simulink model "controller"  (Simulink 8.6)
settings: Solver=FixedStepDiscrete  StartTime=0.0  StopTime=inf  FixedStep=Ts  RelTol=1e-3
InitFcn:
  | initTrqBalancingSeeSaw;
values from neighbouring files (symbols this model uses):
  directionOfOscillation = [0;1;0]    [init.m]
  noOscillationTime = 0    [init.m]
  referenceParams = [0.00  0.1]    [init.m]
  ROBOT_DOF = 23    [init.m]
  seesaw = struct    [init.m]
undefined symbols (not defined in the file or in its folder): bVectorConstraints, CONFIG, ConstraintsMatrix, footSize, gain, LEFT_RIGHT_FOOT_IN_CONTACT, reg, sat
libraries: WBToolboxLibrary x29, WBCLibrary x12, simulink x2
settings Model: Creator=makaveli  LastModifiedBy=DanielePucci
settings DataIOCC: SignalLoggingSaveFormat=Dataset
settings OptimizationCC: ExpressionDepthLimit=128
settings DebuggingCC: UnderspecifiedInitializationDetection=Simplified  MergeDetectMultiDrivingBlocksExec=error  FcnCallInpInsideContextMsg=EnableAllAsError  StateNameClashWarn=none
settings GRTTargetCC: CombineOutputUpdateFcns=on  GRTInterface=off
settings ConfigComp: CovSFcnEnable=off

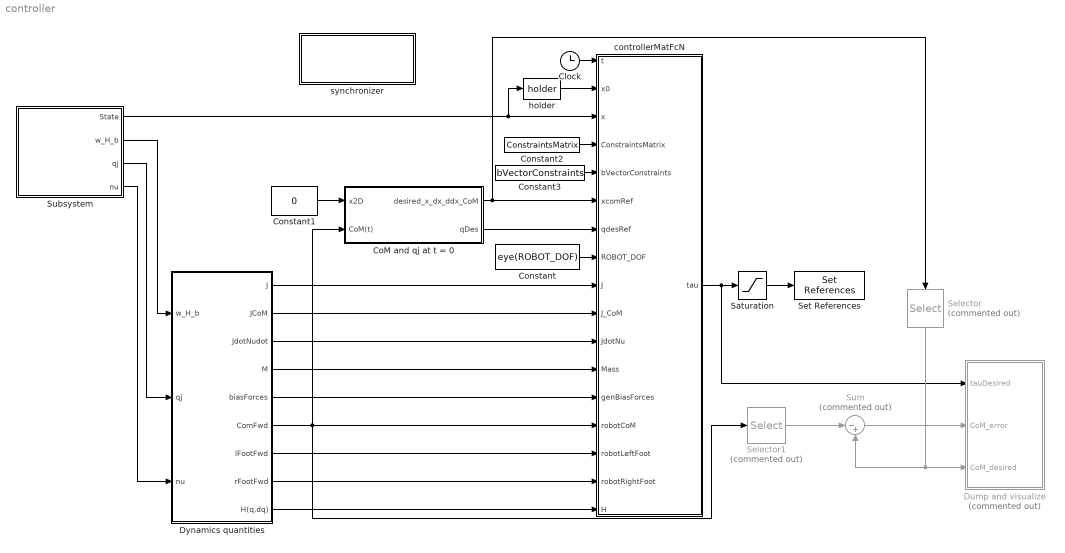
== system controller ==
  Clock : Clock
  CoM and qj at t = 0 : Subsystem  Priority=2
  Constant : Constant  Value=eye(ROBOT_DOF)
  Constant1 : Constant  Value=0
  Constant2 : Constant  Value=ConstraintsMatrix
  Constant3 : Constant  Value=bVectorConstraints
  Dump and visualize : Subsystem  Commented=on
  Dynamics quantities : Subsystem  Priority=3
  Saturation : Saturate  UpperLimit=sat.torque  LowerLimit=-sat.torque
  Selector : Selector  Commented=on  NumberOfDimensions=2  InputPortWidth=3  IndexOptions=Index vector (dialog),Index vector (dialog)  Indices=[1:3],1  OutputSizes=1,1
  Selector1 : Selector  Commented=on  InputPortWidth=7  IndexOptions=Index vector (dialog)  Indices=[1:3]  OutputSizes=1
  Set References : WBToolboxLibrary/wholeBodyActuators/Set References  controlType=Torque  robotName=WBT_robotName  localName=WBT_modelName  wbiFile=WBT_wbiFilename  wbiList=WBT_wbiList
  Subsystem : Subsystem  Priority=1
      mask Display:
      | disp('State');
      | port_label('output',1,'x')
      | port_label('output',2,'w_H_b')
      | port_label('output',3,'q_j')
      | port_label('output',4,'nu')
  Sum : Sum  Commented=on  Inputs=|-+
  controllerMatFcN : MATLAB Function  TreatAsAtomicUnit=on
  "holder " : WBToolboxLibrary/Utilities/holder 
  synchronizer : Subsystem
      mask Display: disp('SYNCHRONIZER')
  wires:
  Clock/1 -> controllerMatFcN/1(t)
  Subsystem/1(State) -> "holder "/1, controllerMatFcN/3(x)
  Subsystem/4(nu) -> Dynamics quantities/3(nu)
  CoM and qj at t = 0/1(desired_x_dx_ddx_CoM) -> Selector/1, controllerMatFcN/6(xcomRef)
  CoM and qj at t = 0/2(qDes) -> controllerMatFcN/7(qdesRef)
  Constant/1 -> controllerMatFcN/8(ROBOT_DOF)
  Dynamics quantities/1(J) -> controllerMatFcN/9(J)
  Dynamics quantities/2(JCoM) -> controllerMatFcN/10(J_CoM)
  Dynamics quantities/3(JdotNudot) -> controllerMatFcN/11(JdotNu)
  Dynamics quantities/4(M) -> controllerMatFcN/12(Mass)
  Dynamics quantities/5(biasForces) -> controllerMatFcN/13(genBiasForces)
  Dynamics quantities/6(ComFwd) -> CoM and qj at t = 0/2(CoM(t)), controllerMatFcN/14(robotCoM), Selector1/1
  Dynamics quantities/7(lFootFwd) -> controllerMatFcN/15(robotLeftFoot)
  Dynamics quantities/8(rFootFwd) -> controllerMatFcN/16(robotRightFoot)
  Dynamics quantities/9(H(q,dq)) -> controllerMatFcN/17(H)
  Saturation/1 -> Set References/1
  controllerMatFcN/1(tau) -> Dump and visualize/1(tauDesired), Saturation/1
  Selector/1 -> Sum/2, Dump and visualize/3(CoM_desired)
  Selector1/1 -> Sum/1
  Sum/1 -> Dump and visualize/2(CoM_error)
  "holder "/1 -> controllerMatFcN/2(x0)
  Subsystem/2(w_H_b) -> Dynamics quantities/1(w_H_b)
  Subsystem/3(qj) -> Dynamics quantities/2(qj)
  Constant1/1 -> CoM and qj at t = 0/1(x2D)
  Constant2/1 -> controllerMatFcN/4(ConstraintsMatrix)
  Constant3/1 -> controllerMatFcN/5(bVectorConstraints)

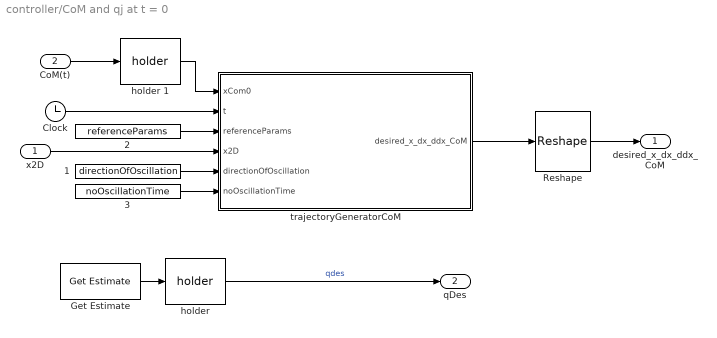
== system controller/CoM and qj at t = 0 ==
  x2D : Inport
  CoM(t) : Inport  Port=2
  "    1" : Constant  Value=directionOfOscillation
  "    2" : Constant  Value=referenceParams
  "    3" : Constant  Value=noOscillationTime
  Clock : Clock
  Get Estimate : WBToolboxLibrary/wholeBodyStates/Get Estimate  estimateType=Joints Position  robotName=WBT_robotName  localName=WBT_modelName  wbiFile=WBT_wbiFilename  wbiList=WBT_wbiList
  Reshape : Reshape  OutputDimensionality=Customize  OutputDimensions=[3,3]
  "holder " : WBToolboxLibrary/Utilities/holder 
  holder 1 : WBToolboxLibrary/Utilities/holder 
  trajectoryGeneratorCoM : MATLAB Function  TreatAsAtomicUnit=on
  desired_x_dx_ddx_CoM : Outport
  qDes : Outport  Port=2
  wires:
  Get Estimate/1 -> "holder "/1
  "holder "/1 -> qDes/1  "qdes"
  holder 1/1 -> trajectoryGeneratorCoM/1(xCom0)
  "    2"/1 -> trajectoryGeneratorCoM/3(referenceParams)
  Clock/1 -> trajectoryGeneratorCoM/2(t)
  "    1"/1 -> trajectoryGeneratorCoM/5(directionOfOscillation)
  "    3"/1 -> trajectoryGeneratorCoM/6(noOscillationTime)
  trajectoryGeneratorCoM/1(desired_x_dx_ddx_CoM) -> Reshape/1
  Reshape/1 -> desired_x_dx_ddx_CoM/1
  x2D/1 -> trajectoryGeneratorCoM/4(x2D)
  CoM(t)/1 -> holder 1/1

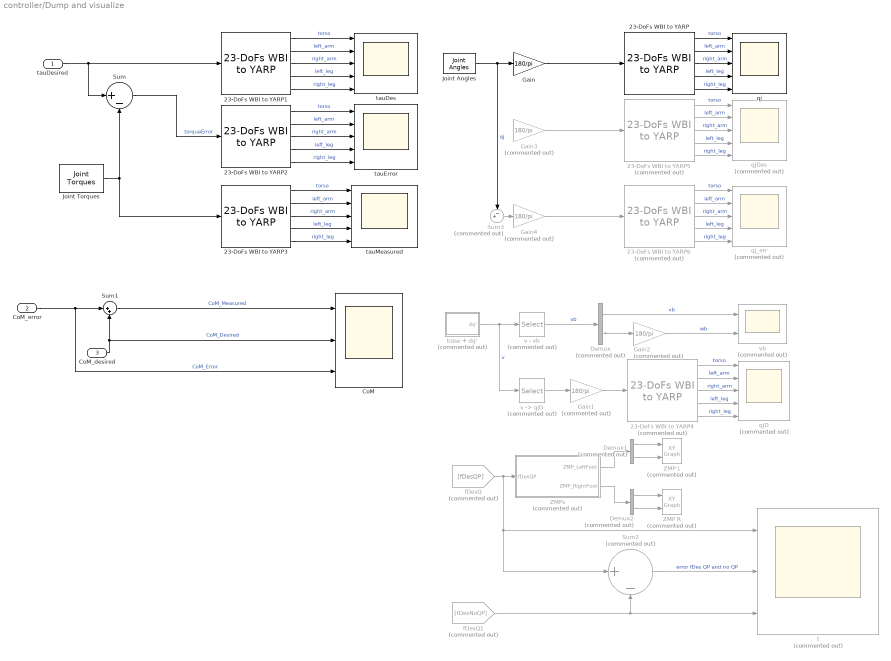
== system controller/Dump and visualize ==
  tauDesired : Inport
  CoM_error : Inport  Port=2
  CoM_desired : Inport  Port=3
  23-DoFs WBI to YARP{,1..3} (4 alike) : WBCLibrary/Utilities/23-DoFs WBI to YARP
  23-DoFs WBI to YARP4 : WBCLibrary/Utilities/23-DoFs WBI to YARP  Commented=on
  23-DoFs WBI to YARP5 : WBCLibrary/Utilities/23-DoFs WBI to YARP  Commented=on
  23-DoFs WBI to YARP6 : WBCLibrary/Utilities/23-DoFs WBI to YARP  Commented=on
  CoM : Scope  NumInputPorts=3
  Demux : Demux  Commented=on  Outputs=2
  Demux1 : Demux  Commented=on  Outputs=2
  Demux2 : Demux  Commented=on  Outputs=2
  Gain : Gain  Gain=180/pi
  Gain{1..4} (4 alike) : Gain  Commented=on  Gain=180/pi
  Joint Angles : WBCLibrary/wholeBodyStates/Joint Angles  robotName=robotName  localName=localName
  Joint Torques : WBCLibrary/wholeBodyStates/Joint Torques  robotName=robotName  localName=localName
  Sum : Sum  Inputs=|+-
  Sum1 : Sum  Inputs=|++
  Sum2 : Sum  Commented=on  Inputs=|+-
  Sum3 : Sum  Commented=on  Inputs=-+|
  ZMP L : simulink/Sinks/XY Graph  Commented=on  xmin=footSize(1,1)  xmax=footSize(1,2)  ymin=footSize(2,1)  ymax=footSize(2,2)  st=-1
  ZMP R : simulink/Sinks/XY Graph  Commented=on  xmin=footSize(1,1)  xmax=footSize(1,2)  ymin=footSize(2,1)  ymax=footSize(2,2)  st=-1
  ZMPs : Subsystem  Commented=on
  base + dq' : Subsystem  Commented=on
  f : Scope  Commented=on  NumInputPorts=3
  fDesQ : From  Commented=on  GotoTag=fDesQP  TagVisibility=global
  fDesQ1 : From  Commented=on  GotoTag=fDesNoQP  TagVisibility=global
  qj : Scope  NumInputPorts=5
  qjD : Scope  Commented=on  NumInputPorts=5
  qjDes : Scope  Commented=on  NumInputPorts=5
  qj_err : Scope  Commented=on  NumInputPorts=5
  tauDes : Scope  NumInputPorts=5
  tauError : Scope  NumInputPorts=5
  tauMeasured : Scope  NumInputPorts=5
  v - vb : Selector  Commented=on  InputPortWidth=ROBOT_DOF+6  IndexOptions=Index vector (dialog)  Indices=[1:6]  OutputSizes=1
  "v -> qjD" : Selector  Commented=on  InputPortWidth=ROBOT_DOF+6  IndexOptions=Index vector (dialog)  Indices=[7:ROBOT_DOF+6]  OutputSizes=1
  vb : Scope  Commented=on  NumInputPorts=2
  wires:
  CoM_error/1 -> CoM/3, Sum1/1  "CoM_Error"
  CoM_desired/1 -> Sum1/2, CoM/2  "CoM_Desired"
  Sum1/1 -> CoM/1  "CoM_Measured"
  base + dq'/1(dq') -> "v -> qjD"/1, v - vb/1  "v"
  Joint Angles/1 -> Sum3/1, Gain/1  "qj"
  Gain/1 -> 23-DoFs WBI to YARP/1
  23-DoFs WBI to YARP/5 -> qj/5  "right_leg"
  23-DoFs WBI to YARP/1 -> qj/1  "torso"
  23-DoFs WBI to YARP/2 -> qj/2  "left_arm"
  23-DoFs WBI to YARP/4 -> qj/4  "left_leg"
  23-DoFs WBI to YARP/3 -> qj/3  "right_arm"
  23-DoFs WBI to YARP4/5 -> qjD/5  "right_leg"
  23-DoFs WBI to YARP4/1 -> qjD/1  "torso"
  23-DoFs WBI to YARP4/2 -> qjD/2  "left_arm"
  23-DoFs WBI to YARP4/4 -> qjD/4  "left_leg"
  23-DoFs WBI to YARP4/3 -> qjD/3  "right_arm"
  "v -> qjD"/1 -> Gain1/1
  v - vb/1 -> Demux/1  "vb"
  Demux/1 -> vb/1  "vb"
  Demux/2 -> Gain2/1
  Gain1/1 -> 23-DoFs WBI to YARP4/1
  Gain2/1 -> vb/2  "wb"
  fDesQ/1 -> Sum2/1, f/1, ZMPs/1(fDesQP)
  ZMPs/1(ZMP_LeftFoot) -> Demux1/1
  ZMPs/2(ZMP_RightFoot) -> Demux2/1
  Demux1/1 -> ZMP L/1
  Demux1/2 -> ZMP L/2
  Demux2/1 -> ZMP R/1
  Demux2/2 -> ZMP R/2
  Sum2/1 -> f/2  "error fDes QP and no QP"
  fDesQ1/1 -> Sum2/2, f/3
  tauDesired/1 -> Sum/1, 23-DoFs WBI to YARP1/1
  Joint Torques/1 -> 23-DoFs WBI to YARP3/1, Sum/2
  23-DoFs WBI to YARP1/5 -> tauDes/5  "right_leg"
  23-DoFs WBI to YARP1/1 -> tauDes/1  "torso"
  23-DoFs WBI to YARP1/2 -> tauDes/2  "left_arm"
  23-DoFs WBI to YARP1/4 -> tauDes/4  "left_leg"
  23-DoFs WBI to YARP1/3 -> tauDes/3  "right_arm"
  23-DoFs WBI to YARP2/5 -> tauError/5  "right_leg"
  23-DoFs WBI to YARP2/1 -> tauError/1  "torso"
  23-DoFs WBI to YARP2/2 -> tauError/2  "left_arm"
  23-DoFs WBI to YARP2/4 -> tauError/4  "left_leg"
  23-DoFs WBI to YARP2/3 -> tauError/3  "right_arm"
  Sum/1 -> 23-DoFs WBI to YARP2/1  "torqueError"
  23-DoFs WBI to YARP3/5 -> tauMeasured/5  "right_leg"
  23-DoFs WBI to YARP3/1 -> tauMeasured/1  "torso"
  23-DoFs WBI to YARP3/2 -> tauMeasured/2  "left_arm"
  23-DoFs WBI to YARP3/4 -> tauMeasured/4  "left_leg"
  23-DoFs WBI to YARP3/3 -> tauMeasured/3  "right_arm"
  ? -> Sum3/2, Gain3/1  "qj_des"
  Gain3/1 -> 23-DoFs WBI to YARP5/1
  23-DoFs WBI to YARP5/5 -> qjDes/5  "right_leg"
  23-DoFs WBI to YARP5/1 -> qjDes/1  "torso"
  23-DoFs WBI to YARP5/2 -> qjDes/2  "left_arm"
  23-DoFs WBI to YARP5/4 -> qjDes/4  "left_leg"
  23-DoFs WBI to YARP5/3 -> qjDes/3  "right_arm"
  Gain4/1 -> 23-DoFs WBI to YARP6/1
  23-DoFs WBI to YARP6/5 -> qj_err/5  "right_leg"
  23-DoFs WBI to YARP6/1 -> qj_err/1  "torso"
  23-DoFs WBI to YARP6/2 -> qj_err/2  "left_arm"
  23-DoFs WBI to YARP6/4 -> qj_err/4  "left_leg"
  23-DoFs WBI to YARP6/3 -> qj_err/3  "right_arm"
  Sum3/1 -> Gain4/1

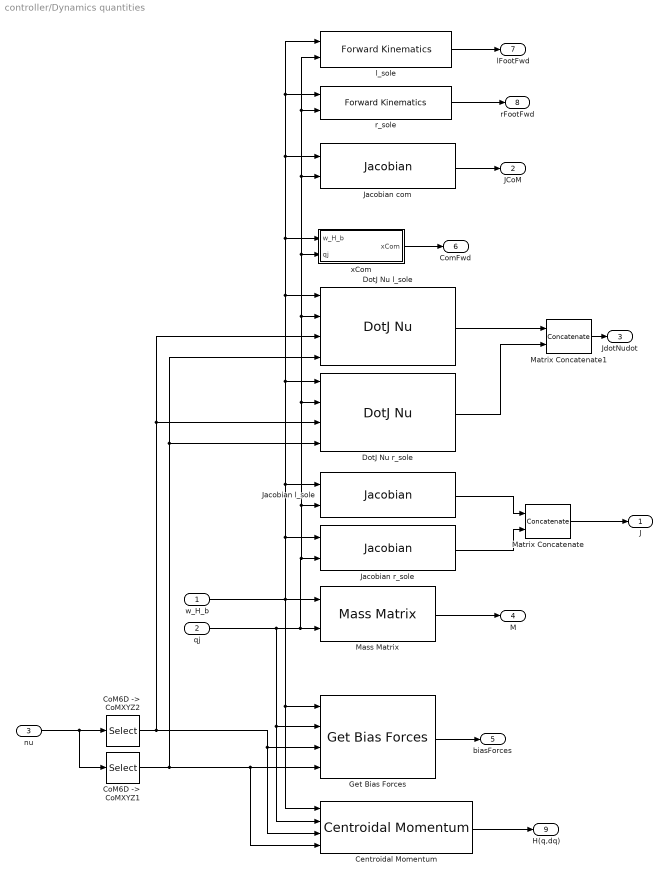
== system controller/Dynamics quantities ==
  w_H_b : Inport
  qj : Inport  Port=2
  nu : Inport  Port=3
  Centroidal Momentum : WBToolboxLibrary/wholeBodyModel/Dynamics/Centroidal Momentum  robotName=WBT_robotName  localName=WBT_modelName  wbiFile=WBT_wbiFilename  wbiList=WBT_wbiList
  "CoM6D ->  CoMXYZ1" : Selector  InputPortWidth=6+ROBOT_DOF  IndexOptions=Index vector (dialog)  Indices=[7:6+ROBOT_DOF]  OutputSizes=1
  "CoM6D ->  CoMXYZ2" : Selector  InputPortWidth=6+ROBOT_DOF  IndexOptions=Index vector (dialog)  Indices=[1 2 3 4 5 6]  OutputSizes=1
  "DotJ Nu l_sole " : WBToolboxLibrary/wholeBodyModel/Jacobians/DotJ Nu  frameName='l_sole'  robotName=WBT_robotName  localName=WBT_modelName  wbiFile=WBT_wbiFilename  wbiList=WBT_wbiList
  "DotJ Nu r_sole " : WBToolboxLibrary/wholeBodyModel/Jacobians/DotJ Nu  frameName='r_sole'  robotName=WBT_robotName  localName=WBT_modelName  wbiFile=WBT_wbiFilename  wbiList=WBT_wbiList
  Get Bias Forces : WBToolboxLibrary/wholeBodyModel/Dynamics/Get Bias Forces  robotName=WBT_robotName  localName=WBT_modelName  wbiFile=WBT_wbiFilename  wbiList=WBT_wbiList  explicitGravity=off
  Jacobian com : WBToolboxLibrary/wholeBodyModel/Jacobians/Jacobian  frameName='com'  robotName=WBT_robotName  localName=WBT_modelName  wbiFile=WBT_wbiFilename  wbiList=WBT_wbiList
  Jacobian l_sole : WBToolboxLibrary/wholeBodyModel/Jacobians/Jacobian  frameName='l_sole'  robotName=WBT_robotName  localName=WBT_modelName  wbiFile=WBT_wbiFilename  wbiList=WBT_wbiList
  Jacobian r_sole : WBToolboxLibrary/wholeBodyModel/Jacobians/Jacobian  frameName='r_sole'  robotName=WBT_robotName  localName=WBT_modelName  wbiFile=WBT_wbiFilename  wbiList=WBT_wbiList
  Mass Matrix : WBToolboxLibrary/wholeBodyModel/Dynamics/Mass Matrix  robotName=WBT_robotName  localName=WBT_modelName  wbiFile=WBT_wbiFilename  wbiList=WBT_wbiList
  Matrix Concatenate : Concatenate  Mode=Multidimensional array
  Matrix Concatenate1 : Concatenate  Mode=Multidimensional array
  l_sole : WBToolboxLibrary/wholeBodyModel/Kinematics/Forward Kinematics  frameName='l_sole'  robotName=WBT_robotName  localName=WBT_modelName  wbiFile=WBT_wbiFilename  wbiList=WBT_wbiList
  r_sole : WBToolboxLibrary/wholeBodyModel/Kinematics/Forward Kinematics  frameName='r_sole'  robotName=WBT_robotName  localName=WBT_modelName  wbiFile=WBT_wbiFilename  wbiList=WBT_wbiList
  xCom : Subsystem
  J : Outport
  JCoM : Outport  Port=2
  JdotNudot : Outport  Port=3
  M : Outport  Port=4
  biasForces : Outport  Port=5
  ComFwd : Outport  Port=6
  lFootFwd : Outport  Port=7
  rFootFwd : Outport  Port=8
  H(q,dq) : Outport  Port=9
  wires:
  Get Bias Forces/1 -> biasForces/1
  Matrix Concatenate1/1 -> JdotNudot/1
  Jacobian r_sole/1 -> Matrix Concatenate/2
  l_sole/1 -> lFootFwd/1
  xCom/1(xCom) -> ComFwd/1
  r_sole/1 -> rFootFwd/1
  Matrix Concatenate/1 -> J/1
  Jacobian l_sole/1 -> Matrix Concatenate/1
  Jacobian com/1 -> JCoM/1
  w_H_b/1 -> Jacobian r_sole/1, "DotJ Nu r_sole "/1, r_sole/1, l_sole/1, Jacobian com/1, xCom/1(w_H_b), "DotJ Nu l_sole "/1, Jacobian l_sole/1, Mass Matrix/1, Centroidal Momentum/1, Get Bias Forces/1
  qj/1 -> r_sole/2, l_sole/2, Jacobian com/2, xCom/2(qj), "DotJ Nu l_sole "/2, "DotJ Nu r_sole "/2, Jacobian l_sole/2, Jacobian r_sole/2, Mass Matrix/2, Get Bias Forces/2, Centroidal Momentum/2
  "CoM6D ->  CoMXYZ2"/1 -> "DotJ Nu r_sole "/3, "DotJ Nu l_sole "/3, Centroidal Momentum/3, Get Bias Forces/3
  "CoM6D ->  CoMXYZ1"/1 -> "DotJ Nu r_sole "/4, "DotJ Nu l_sole "/4, Get Bias Forces/4, Centroidal Momentum/4
  nu/1 -> "CoM6D ->  CoMXYZ1"/1, "CoM6D ->  CoMXYZ2"/1
  Centroidal Momentum/1 -> H(q,dq)/1
  Mass Matrix/1 -> M/1
  "DotJ Nu l_sole "/1 -> Matrix Concatenate1/1
  "DotJ Nu r_sole "/1 -> Matrix Concatenate1/2

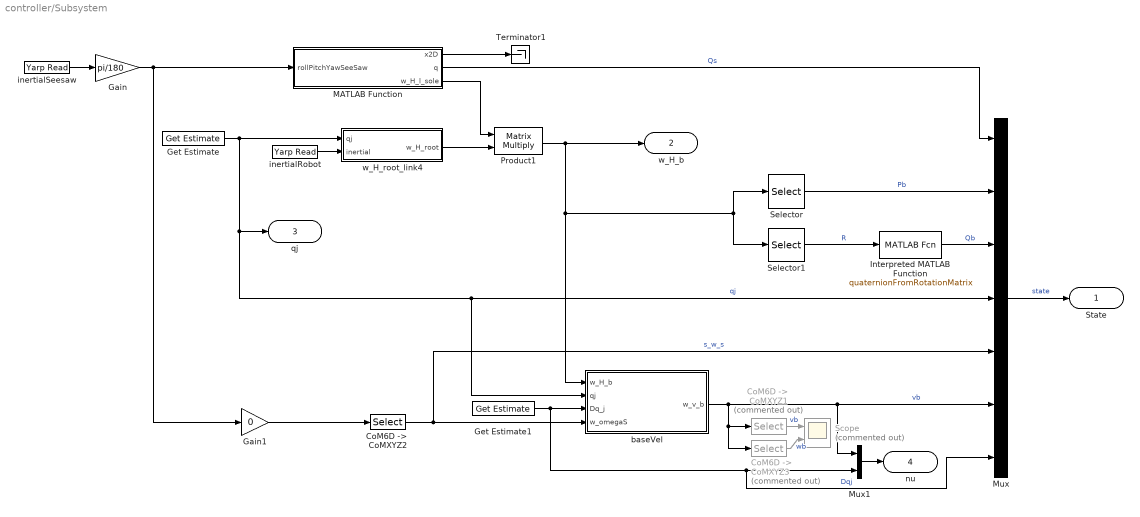
== system controller/Subsystem ==
  "CoM6D ->  CoMXYZ1" : Selector  Commented=on  InputPortWidth=6  IndexOptions=Index vector (dialog)  Indices=[1 2 3]  OutputSizes=1
  "CoM6D ->  CoMXYZ2" : Selector  InputPortWidth=12  IndexOptions=Index vector (dialog)  Indices=[7 8 9]  OutputSizes=1
  "CoM6D ->  CoMXYZ3" : Selector  Commented=on  InputPortWidth=6  IndexOptions=Index vector (dialog)  Indices=[4 5 6]  OutputSizes=1
  Gain : Gain  Gain=pi/180
  Gain1 : Gain  Gain=0
  Get Estimate : WBToolboxLibrary/wholeBodyStates/Get Estimate  estimateType=Joints Position  robotName=WBT_robotName  localName=WBT_modelName  wbiFile=WBT_wbiFilename  wbiList=WBT_wbiList
  Get Estimate1 : WBToolboxLibrary/wholeBodyStates/Get Estimate  estimateType=Joints Velocity  robotName=WBT_robotName  localName=WBT_modelName  wbiFile=WBT_wbiFilename  wbiList=WBT_wbiList
  Interpreted MATLAB Function : MATLABFcn  MATLABFcn=quaternionFromRotationMatrix  OutputDimensions=4
  MATLAB Function : MATLAB Function  Priority=10  TreatAsAtomicUnit=on
  Mux : Mux  Inputs=7
  Mux1 : Mux  Inputs=2
  Product1 : Product  Priority=19  Multiplication=Matrix(*)
  Scope : Scope  Commented=on  NumInputPorts=2
  Selector : Selector  NumberOfDimensions=2  InputPortWidth=3  IndexOptions=Index vector (dialog),Index vector (dialog)  Indices=[1:3],4  OutputSizes=1,1
  Selector1 : Selector  NumberOfDimensions=2  InputPortWidth=3  IndexOptions=Index vector (dialog),Index vector (dialog)  Indices=[1:3],[1:3]  OutputSizes=1,1
  Terminator1 : Terminator
  baseVel : Subsystem
  inertialRobot : WBToolboxLibrary/Utilities/Yarp Read  portName='/icub/inertial'  signalSize=12  blocking=off  timestamp=off  autoconnect=on  errorOnConnection=off
  inertialSeesaw : WBToolboxLibrary/Utilities/Yarp Read  portName=seesaw_inertial  signalSize=12  blocking=off  timestamp=off  autoconnect=on  errorOnConnection=on
  w_H_root_link4 : Subsystem  mask{link_name='l_sole'}
      mask prompts: link_name "link name"
      mask help:
      | This block evaluates the homogeneous transformation between the world and the root link, i.e. ^wH_b. It assumes that the link specified by the variable 'link_name' has a constant position
      | w.r.t. an inertial frame, but it can rotate arbitrarily. This rotation is retrived from the IMU sensor.
      mask Display:
      | str = strrep(link_name, '_','\_');
      | port_label('output',1,['{}^{',str '}H_{root}'],'texmode','on')
      | clear str;
      | 
      | port_label('input',1,'q_j','texmode','on')
      | 
      | port_label('input',2,'inertial','texmode','on')
  State : Outport
  w_H_b : Outport  Port=2
  qj : Outport  Port=3
  nu : Outport  Port=4
  wires:
  Get Estimate1/1 -> Mux/7, Mux1/2, baseVel/3(Dq_j)  "Dqj"
  Get Estimate/1 -> w_H_root_link4/1(qj), qj/1, baseVel/2(qj), Mux/4  "qj"
  Mux/1 -> State/1  "state"
  Selector/1 -> Mux/2  "Pb"
  Selector1/1 -> Interpreted MATLAB Function/1  "R"
  Interpreted MATLAB Function/1 -> Mux/3  "Qb"
  Mux1/1 -> nu/1
  baseVel/1(w_v_b) -> Mux1/1, Mux/6, "CoM6D ->  CoMXYZ3"/1, "CoM6D ->  CoMXYZ1"/1  "vb"
  MATLAB Function/2(q) -> Mux/1  "Qs"
  Product1/1 -> w_H_b/1, baseVel/1(w_H_b), Selector1/1, Selector/1
  MATLAB Function/3(w_H_l_sole) -> Product1/1
  MATLAB Function/1(x2D) -> Terminator1/1
  "CoM6D ->  CoMXYZ2"/1 -> Mux/5, baseVel/4(w_omegaS)  "s_w_s"
  inertialSeesaw/1 -> Gain/1
  Gain/1 -> Gain1/1, MATLAB Function/1(rollPitchYawSeeSaw)
  "CoM6D ->  CoMXYZ1"/1 -> Scope/1  "vb"
  "CoM6D ->  CoMXYZ3"/1 -> Scope/2  "wb"
  Gain1/1 -> "CoM6D ->  CoMXYZ2"/1
  inertialRobot/1 -> w_H_root_link4/2(inertial)
  w_H_root_link4/1(w_H_root) -> Product1/2

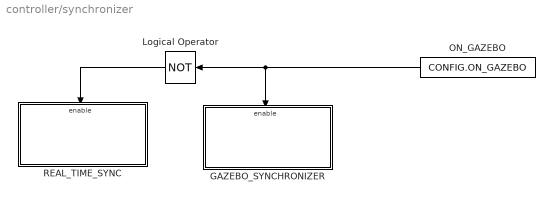
== system controller/synchronizer ==
  GAZEBO_SYNCHRONIZER : Subsystem
  Logical Operator : Logic  Operator=NOT  AllPortsSameDT=off  OutDataTypeStr=boolean
  "ON_GAZEBO " : Constant  Value=CONFIG.ON_GAZEBO
  REAL_TIME_SYNC : Subsystem
  wires:
  Logical Operator/1 -> REAL_TIME_SYNC/Enable
  "ON_GAZEBO "/1 -> GAZEBO_SYNCHRONIZER/Enable, Logical Operator/1

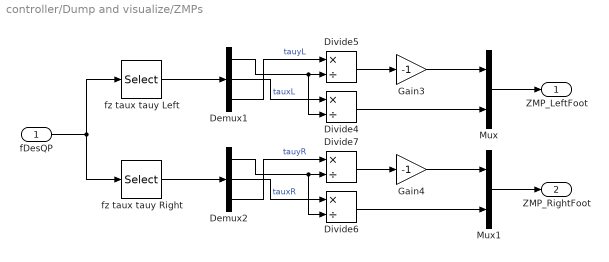
== system controller/Dump and visualize/ZMPs ==
  fDesQP : Inport
  Demux1 : Demux  Outputs=3
  Demux2 : Demux  Outputs=3
  Divide{4..7} (4 alike) : Product  Inputs=*/
  Gain3 : Gain  Gain=-1
  Gain4 : Gain  Gain=-1
  Mux : Mux  Inputs=2
  Mux1 : Mux  Inputs=2
  fz taux tauy Left : Selector  InputPortWidth=12  IndexOptions=Index vector (dialog)  Indices=[3 4 5]  OutputSizes=1
  fz taux tauy Right : Selector  InputPortWidth=12  IndexOptions=Index vector (dialog)  Indices=[9 10 11]  OutputSizes=1
  ZMP_LeftFoot : Outport
  ZMP_RightFoot : Outport  Port=2
  wires:
  fz taux tauy Left/1 -> Demux1/1
  Demux1/1 -> Divide4/2, Divide5/2
  Divide7/1 -> Gain4/1
  Divide4/1 -> Mux/2
  Divide5/1 -> Gain3/1
  fz taux tauy Right/1 -> Demux2/1
  Demux2/1 -> Divide6/2, Divide7/2
  fDesQP/1 -> fz taux tauy Left/1, fz taux tauy Right/1
  Gain3/1 -> Mux/1
  Mux/1 -> ZMP_LeftFoot/1
  Divide6/1 -> Mux1/2
  Gain4/1 -> Mux1/1
  Mux1/1 -> ZMP_RightFoot/1
  Demux1/2 -> Divide4/1  "tauxL"
  Demux1/3 -> Divide5/1  "tauyL"
  Demux2/2 -> Divide6/1  "tauxR"
  Demux2/3 -> Divide7/1  "tauyR"

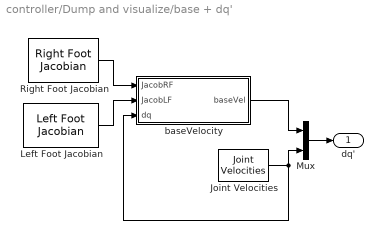
== system controller/Dump and visualize/base + dq' ==
  Joint Velocities : WBCLibrary/wholeBodyStates/Joint Velocities  robotName=robotName  localName=localName
  Left Foot Jacobian : WBCLibrary/wholeBodyModel/Jacobians/Left Foot Jacobian  robotName=robotName  localName=localName
  Mux : Mux  Inputs=2
  Right Foot Jacobian : WBCLibrary/wholeBodyModel/Jacobians/Right Foot Jacobian  robotName=robotName  localName=localName
  baseVelocity : Subsystem  AncestorBlock=WBCLibrary/Utilities/baseVelocity  mask(baseVelocity){}
      mask help: This block computes the velocity of the floating base of a bipedal robot
  dq' : Outport
  wires:
  Left Foot Jacobian/1 -> baseVelocity/2(JacobLF)
  Right Foot Jacobian/1 -> baseVelocity/1(JacobRF)
  baseVelocity/1(baseVel) -> Mux/1
  Joint Velocities/1 -> baseVelocity/3(dq), Mux/2
  Mux/1 -> dq'/1

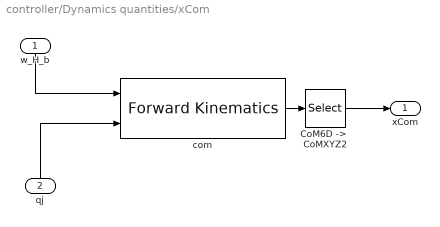
== system controller/Dynamics quantities/xCom ==
  w_H_b : Inport
  qj : Inport  Port=2
  "CoM6D ->  CoMXYZ2" : Selector  NumberOfDimensions=2  InputPortWidth=7  IndexOptions=Index vector (dialog),Index vector (dialog)  Indices=[1 2 3],[4]  OutputSizes=1,1
  com : WBToolboxLibrary/wholeBodyModel/Kinematics/Forward Kinematics  frameName='com'  robotName=WBT_robotName  localName=WBT_modelName  wbiFile=WBT_wbiFilename  wbiList=WBT_wbiList
  xCom : Outport
  wires:
  qj/1 -> com/2
  "CoM6D ->  CoMXYZ2"/1 -> xCom/1
  com/1 -> "CoM6D ->  CoMXYZ2"/1
  w_H_b/1 -> com/1

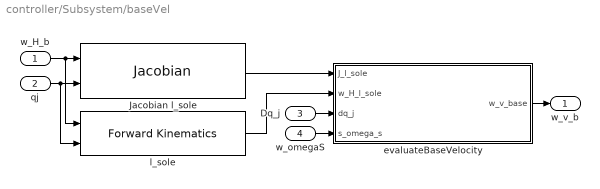
== system controller/Subsystem/baseVel ==
  w_H_b : Inport
  qj : Inport  Port=2
  Dq_j : Inport  Port=3
  w_omegaS : Inport  Port=4
  Jacobian l_sole : WBToolboxLibrary/wholeBodyModel/Jacobians/Jacobian  frameName='l_sole'  robotName=WBT_robotName  localName=WBT_modelName  wbiFile=WBT_wbiFilename  wbiList=WBT_wbiList
  evaluateBaseVelocity : MATLAB Function  Priority=10  TreatAsAtomicUnit=on
  l_sole : WBToolboxLibrary/wholeBodyModel/Kinematics/Forward Kinematics  frameName='l_sole'  robotName=WBT_robotName  localName=WBT_modelName  wbiFile=WBT_wbiFilename  wbiList=WBT_wbiList
  w_v_b : Outport
  wires:
  l_sole/1 -> evaluateBaseVelocity/2(w_H_l_sole)
  w_H_b/1 -> l_sole/1, Jacobian l_sole/1
  evaluateBaseVelocity/1(w_v_base) -> w_v_b/1
  w_omegaS/1 -> evaluateBaseVelocity/4(s_omega_s)
  qj/1 -> l_sole/2, Jacobian l_sole/2
  Dq_j/1 -> evaluateBaseVelocity/3(dq_j)
  Jacobian l_sole/1 -> evaluateBaseVelocity/1(J_l_sole)

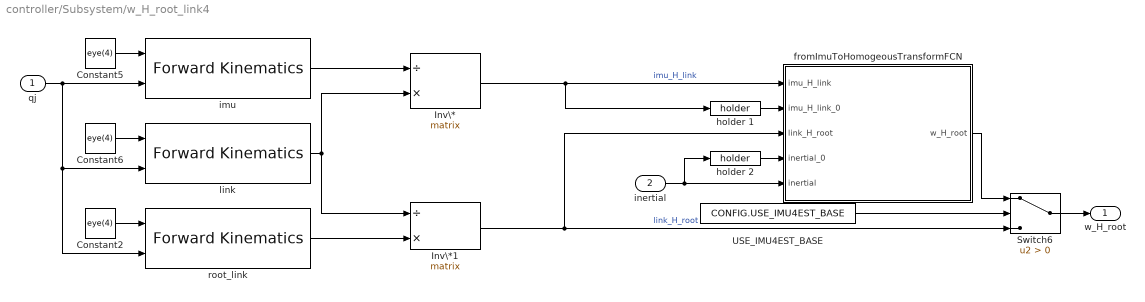
== system controller/Subsystem/w_H_root_link4 ==
  qj : Inport
  inertial : Inport  Port=2
  Constant2 : Constant  Value=eye(4)
  Constant5 : Constant  Value=eye(4)
  Constant6 : Constant  Value=eye(4)
  Inv\* : Product  Inputs=/*  Multiplication=Matrix(*)
  Inv\*1 : Product  Inputs=/*  Multiplication=Matrix(*)
  Switch6 : Switch  Criteria=u2 > Threshold
  USE_IMU4EST_BASE : Constant  Value=CONFIG.USE_IMU4EST_BASE
  fromImuToHomogeousTransformFCN : MATLAB Function  TreatAsAtomicUnit=on
  holder 1 : WBToolboxLibrary/Utilities/holder 
  holder 2 : WBToolboxLibrary/Utilities/holder 
  imu : WBToolboxLibrary/wholeBodyModel/Kinematics/Forward Kinematics  frameName='imu_frame'  robotName=WBT_robotName  localName=WBT_modelName  wbiFile=WBT_wbiFilename  wbiList=WBT_wbiList
  link : WBToolboxLibrary/wholeBodyModel/Kinematics/Forward Kinematics  frameName=link_name  robotName=WBT_robotName  localName=WBT_modelName  wbiFile=WBT_wbiFilename  wbiList=WBT_wbiList
  root_link : WBToolboxLibrary/wholeBodyModel/Kinematics/Forward Kinematics  frameName='root_link'  robotName=WBT_robotName  localName=WBT_modelName  wbiFile=WBT_wbiFilename  wbiList=WBT_wbiList
  w_H_root : Outport
  wires:
  Constant5/1 -> imu/1
  Inv\*/1 -> holder 1/1, fromImuToHomogeousTransformFCN/1(imu_H_link)  "imu_H_link"
  imu/1 -> Inv\*/1
  Constant6/1 -> link/1
  Inv\*1/1 -> Switch6/3, fromImuToHomogeousTransformFCN/3(link_H_root)  "link_H_root"
  link/1 -> Inv\*/2, Inv\*1/1
  inertial/1 -> holder 2/1, fromImuToHomogeousTransformFCN/5(inertial)
  Switch6/1 -> w_H_root/1
  USE_IMU4EST_BASE/1 -> Switch6/2
  fromImuToHomogeousTransformFCN/1(w_H_root) -> Switch6/1
  Constant2/1 -> root_link/1
  qj/1 -> root_link/2, link/2, imu/2
  root_link/1 -> Inv\*1/2
  holder 1/1 -> fromImuToHomogeousTransformFCN/2(imu_H_link_0)
  holder 2/1 -> fromImuToHomogeousTransformFCN/4(inertial_0)

== system controller/synchronizer/GAZEBO_SYNCHRONIZER ==
  Enable : EnablePort
  Simulator Synchronizer : WBToolboxLibrary/Utilities/Simulator Synchronizer  period=CONFIG.TS  serverPortName='/clock/rpc'  clientPortName='/WBT_synchronizer/rpc:o'

== system controller/synchronizer/REAL_TIME_SYNC ==
  Enable : EnablePort
  Real Time Synchronizer : WBToolboxLibrary/Utilities/Real Time Synchronizer  period=CONFIG.TS

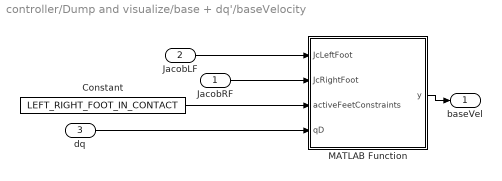
== system controller/Dump and visualize/base + dq'/baseVelocity ==
  JacobRF : Inport
  JacobLF : Inport  Port=2
  dq : Inport  Port=3
  Constant : Constant  Value=LEFT_RIGHT_FOOT_IN_CONTACT
  MATLAB Function : MATLAB Function  TreatAsAtomicUnit=on
  baseVel : Outport
  wires:
  JacobLF/1 -> MATLAB Function/1(JcLeftFoot)
  JacobRF/1 -> MATLAB Function/2(JcRightFoot)
  MATLAB Function/1(y) -> baseVel/1
  dq/1 -> MATLAB Function/4(qD)
  Constant/1 -> MATLAB Function/3(activeFeetConstraints)

== matlab function controllerMatFcN ==
  data: tau output double; t input double; x0 input double; x input double; ConstraintsMatrix input double; bVectorConstraints input double; gain parameter double; reg parameter double; xcomRef input double; qdesRef input double; seesaw parameter double; ROBOT_DOF input double; J input double; J_CoM input double; JdotNu input double; Mass input double; genBiasForces input double; robotCoM input double; robotLeftFoot input double; robotRightFoot input double; H input double; CONFIG parameter double
 function tau = fcn(t, x0,x,ConstraintsMatrix,bVectorConstraints, ...
    gain, reg, ...
    xcomRef, qdesRef,  ...
    seesaw, ROBOT_DOF,...
    J, J_CoM, JdotNu, Mass, genBiasForces, robotCoM, robotLeftFoot, robotRightFoot,H,CONFIG)
%#codegen

persistent lFootCentreDistance rFootCentreDistance;

tau                       = zeros(size(ROBOT_DOF, 1), 1);
robot                     = struct;
robot.dofs                = size(ROBOT_DOF, 1);

if isempty(lFootCentreDistance)
    lFootCentreDistance   =  0.1;%robotLeftFoot(2);
    rFootCentreDistance   = -0.1;%robotRightFoot(2);
end

robotWBM.Mass             = Mass;
robotWBM.J                = J;
robotWBM.JdotNu           = JdotNu;
robotWBM.genBiasForces    = genBiasForces;
robotWBM.fwdkin.com       = robotCoM;
robotWBM.fwdkin.l_sole    = robotLeftFoot(1:3,4);
robotWBM.fwdkin.r_sole    = robotRightFoot(1:3,4);
robotWBM.fwdkin.RotMl_sole= robotLeftFoot(1:3,1:3);
robotWBM.fwdkin.RotMr_sole= robotRightFoot(1:3,1:3);

robot.lFootCentreDistance = lFootCentreDistance;
robot.rFootCentreDistance = rFootCentreDistance;

controlParams.gains                = gain;
controlParams.references.qDes      = qdesRef;
controlParams.references.xcomDes   = xcomRef(:,1);
controlParams.references.DxcomDes  = xcomRef(:,2);
controlParams.references.DDxcomDes = xcomRef(:,3);

model = struct('robot', robot, 'seesaw', seesaw);

tau(:) = balancingControlSeeSaw(t, x,ConstraintsMatrix,bVectorConstraints,J_CoM,H,controlParams, model, robotWBM,reg,CONFIG,gain);

== matlab function Subsystem/MATLAB Function ==
  data: x2D output double; q output double; w_H_l_sole output double; rollPitchYawSeeSaw input double; seesaw parameter double
function [x2D,q,w_H_l_sole] = fcn(rollPitchYawSeeSaw,seesaw)
%#codegen
%%Must check that euler angles are x-y-z

q = zeros(4,1);

w_R_s      = rotz(rollPitchYawSeeSaw(3))*roty(rollPitchYawSeeSaw(2))*rotx(rollPitchYawSeeSaw(1));

q(1:4) = quaternionFromRotationMatrix(w_R_s);
e3 = [0;0;1];


leftFoot_s     = [0;  0.1; seesaw.top];

OC = [0;-seesaw.rho*(rollPitchYawSeeSaw(1)/180)*pi;seesaw.rho]; 
CL = w_R_s*(leftFoot_s-seesaw.delta*e3  );    

P_l = OC + CL;
w_H_l_sole = [w_R_s,     P_l;
              zeros(1,3),  1];
          
alpha = 0.0;
mR = 30;          
theta = rollPitchYawSeeSaw(1)*(pi/180);
x2D = -(theta*seesaw.rho*mR + seesaw.delta * seesaw.mass * sin(theta))/mR + alpha*theta;

== matlab function CoM and qj at t = 0/trajectoryGeneratorCoM ==
  data: desired_x_dx_ddx_CoM output double; xCom0 input double; t input double; referenceParams input double; x2D input double; directionOfOscillation input double; noOscillationTime input double
function desired_x_dx_ddx_CoM   = fcn(xCom0,t,referenceParams,x2D,directionOfOscillation,noOscillationTime)
%#codegen


if t > noOscillationTime
    A = referenceParams(1);
else
    A = 0;
end
f = referenceParams(2);

xcomDes    = xCom0 + A*sin(2*pi*f*t)*directionOfOscillation;
% xcomDes(1) =  xcomDes(1) + 0.01;
xDcomDes   =         A*2*pi*f*cos(2*pi*f*t)*directionOfOscillation;
xDDcomDes  =        -A*(2*pi*f)^2*sin(2*pi*f*t)*directionOfOscillation;
xcomDes(2) =        x2D + xCom0(2);
desired_x_dx_ddx_CoM = [xcomDes;xDcomDes;xDDcomDes];

== matlab function Subsystem/baseVel/evaluateBaseVelocity ==
  data: w_v_base output double; J_l_sole input double; w_H_l_sole input double; dq_j input double; s_omega_s input double; model parameter double
function w_v_base  = fcn(J_l_sole, w_H_l_sole,dq_j, s_omega_s, model)
%#codegen


w_R_s          = w_H_l_sole(1:3,1:3);

w_omega_s      = w_R_s*s_omega_s;

e3 = [0;0;1];
w_r            = model.seesaw.delta * w_R_s * e3 - model.seesaw.rho * e3 ; 

s_s_l          = [0; model.robot.lFootCentreDistance; model.seesaw.top];

w_s_l          = w_R_s * s_s_l;
 

 
w_v_l_sole     = [Sf(w_r - w_s_l)*w_omega_s; w_omega_s];

 
w_v_base       = J_l_sole(1:6,1:6)\(w_v_l_sole - J_l_sole(1:6,7:end)*dq_j);

== matlab function Dump and visualize/base + dq'/baseVelocity/MATLAB Function ==
  data: JcLeftFoot input double; JcRightFoot input double; activeFeetConstraints input double; y output double; qD input double
function y = fcn(JcLeftFoot,JcRightFoot,activeFeetConstraints,qD)
%#codegen
if sum(activeFeetConstraints) == 2
    Jc = [JcLeftFoot;JcRightFoot];
else
    Jc = JcLeftFoot;
end
y = -pinv(Jc(:,1:6))*Jc(:,7:end)*qD;

== matlab function Subsystem/w_H_root_link4/fromImuToHomogeousTransformFCN ==
  data: imu_H_link input double; imu_H_link_0 input double; link_H_root input double; inertial_0 input double; inertial input double; w_H_root output double; CONFIG parameter double
function w_H_root = fromBaseToWorldWithImuFCN(imu_H_link,imu_H_link_0,link_H_root,inertial_0,inertial,CONFIG)
%#codegen
w_H_root = fromBaseToWorldWithImu(imu_H_link,imu_H_link_0,link_H_root,inertial_0,inertial,CONFIG);
